simulink model "DWT_opt_fixed_point"  (R2022b)
settings: Solver=VariableStepAuto  StartTime=0.0  StopTime=st*279+st*length(signalx)  RelTol=1e-3
undefined symbols (not defined in the file): st, xc7z020clg484
libraries: hdlBasic x690, vmcUtilities x1
(part 3 of 3)

== system DWT_opt_fixed_point/axis_dwt/Syn_cell2/R_LO ==
  In1 : Inport
  AddSub{,1..6} (7 alike) : hdlBasic/AddSub  mode=Addition  use_carryin=off  use_carryout=off  en=off  latency=0  precision=User Defined  arith_type=Unsigned  n_bits=18  bin_pt=16  quantization=Truncate  overflow=Wrap  use_behavioral_HDL=off  hw_selection=Fabric  pipelined=off  XmcBlockStatus=1  maskContainerNames=tabcontainer1  block_type=addsub  block_config=sysgen:Addsub_config
  Constant : hdlBasic/Constant  const=0.23037781330885523  gui_display_data_type=Fixed-point  arith_type=Signed (2's comp)  n_bits=16  bin_pt=14  preci_type=Single  exp_width=8  frac_width=24  explicit_period=off  period=1  XmcBlockStatus=1  maskContainerNames=tabcontainer1  block_type=constant  block_config=sysgen:Constant_config
  Constant1 : hdlBasic/Constant  const=0.7148465705525415  gui_display_data_type=Fixed-point  arith_type=Signed (2's comp)  n_bits=16  bin_pt=14  preci_type=Single  exp_width=8  frac_width=24  explicit_period=off  period=1  XmcBlockStatus=1  maskContainerNames=tabcontainer1  block_type=constant  block_config=sysgen:Constant_config
  Constant2 : hdlBasic/Constant  const=0.6308807679295904  gui_display_data_type=Fixed-point  arith_type=Signed (2's comp)  n_bits=16  bin_pt=14  preci_type=Single  exp_width=8  frac_width=24  explicit_period=off  period=1  XmcBlockStatus=1  maskContainerNames=tabcontainer1  block_type=constant  block_config=sysgen:Constant_config
  Constant3 : hdlBasic/Constant  const=-0.02798376941698385  gui_display_data_type=Fixed-point  arith_type=Signed (2's comp)  n_bits=16  bin_pt=14  preci_type=Single  exp_width=8  frac_width=24  explicit_period=off  period=1  XmcBlockStatus=1  maskContainerNames=tabcontainer1  block_type=constant  block_config=sysgen:Constant_config
  Constant4 : hdlBasic/Constant  const=-0.18703481171888114  gui_display_data_type=Fixed-point  arith_type=Signed (2's comp)  n_bits=16  bin_pt=14  preci_type=Single  exp_width=8  frac_width=24  explicit_period=off  period=1  XmcBlockStatus=1  maskContainerNames=tabcontainer1  block_type=constant  block_config=sysgen:Constant_config
  Constant5 : hdlBasic/Constant  const=0.030841381835986965  gui_display_data_type=Fixed-point  arith_type=Signed (2's comp)  n_bits=16  bin_pt=14  preci_type=Single  exp_width=8  frac_width=24  explicit_period=off  period=1  XmcBlockStatus=1  maskContainerNames=tabcontainer1  block_type=constant  block_config=sysgen:Constant_config
  Constant6 : hdlBasic/Constant  const=0.032883011666982945  gui_display_data_type=Fixed-point  arith_type=Signed (2's comp)  n_bits=16  bin_pt=14  preci_type=Single  exp_width=8  frac_width=24  explicit_period=off  period=1  XmcBlockStatus=1  maskContainerNames=tabcontainer1  block_type=constant  block_config=sysgen:Constant_config
  Constant7 : hdlBasic/Constant  const=-0.010597401784997278  gui_display_data_type=Fixed-point  arith_type=Signed (2's comp)  n_bits=16  bin_pt=14  preci_type=Single  exp_width=8  frac_width=24  explicit_period=off  period=1  XmcBlockStatus=1  maskContainerNames=tabcontainer1  block_type=constant  block_config=sysgen:Constant_config
  Delay{,1..6} (7 alike) : hdlBasic/Delay  rst=off  en=off  latency=1  reg_retiming=off  XmcBlockStatus=1  maskContainerNames=group1  block_type=delay  block_config=sysgen:Delay_config
  Mult{,1..7} (8 alike) : hdlBasic/Mult  precision=User Defined  arith_type="Signed  (2's comp)"  n_bits=18  bin_pt=16  quantization=Truncate  overflow=Wrap  en=off  latency=0  use_behavioral_HDL=off  opt=Speed  use_embedded=on  optimum_pipeline=off  pipeline=on  use_rpm=on  placement_style=Triangular  XmcBlockStatus=1  maskContainerNames=group1  block_type=mult  block_config=sysgen:Mult_config  block_width=598  block_height=876
  Out1 : Outport
  wires:
  Delay3/1 -> Mult4/2, Delay4/1
  Mult2/1 -> AddSub1/1
  In1/1 -> Mult/2, Delay/1
  Constant6/1 -> Mult6/1
  Delay5/1 -> Mult6/2, Delay6/1
  Constant7/1 -> Mult7/1
  Delay1/1 -> Mult2/2, Delay2/1
  Delay/1 -> Mult1/2, Delay1/1
  AddSub6/1 -> Out1/1
  Delay2/1 -> Mult3/2, Delay3/1
  AddSub3/1 -> AddSub4/2
  Delay6/1 -> Mult7/2
  Mult3/1 -> AddSub2/1
  Constant5/1 -> Mult5/1
  AddSub/1 -> AddSub1/2
  Delay4/1 -> Mult5/2, Delay5/1
  Constant2/1 -> Mult2/1
  Mult7/1 -> AddSub6/1
  Mult1/1 -> AddSub/1
  Mult6/1 -> AddSub5/1
  AddSub4/1 -> AddSub5/2
  Mult4/1 -> AddSub3/1
  AddSub2/1 -> AddSub3/2
  Constant3/1 -> Mult3/1
  Constant/1 -> Mult/1
  Mult5/1 -> AddSub4/1
  AddSub1/1 -> AddSub2/2
  Constant4/1 -> Mult4/1
  Mult/1 -> AddSub/2
  AddSub5/1 -> AddSub6/2
  Constant1/1 -> Mult1/1

== system DWT_opt_fixed_point/axis_dwt/Syn_cell3/R_HI ==
  In1 : Inport
  AddSub{,1..6} (7 alike) : hdlBasic/AddSub  mode=Addition  use_carryin=off  use_carryout=off  en=off  latency=0  precision=User Defined  arith_type=Unsigned  n_bits=18  bin_pt=16  quantization=Truncate  overflow=Wrap  use_behavioral_HDL=off  hw_selection=Fabric  pipelined=off  XmcBlockStatus=1  maskContainerNames=tabcontainer1  block_type=addsub  block_config=sysgen:Addsub_config
  Constant : hdlBasic/Constant  const=-0.010597401784997278  gui_display_data_type=Fixed-point  arith_type=Signed (2's comp)  n_bits=16  bin_pt=14  preci_type=Single  exp_width=8  frac_width=24  explicit_period=off  period=1  XmcBlockStatus=1  maskContainerNames=tabcontainer1  block_type=constant  block_config=sysgen:Constant_config
  Constant1 : hdlBasic/Constant  const=-0.032883011666982945  gui_display_data_type=Fixed-point  arith_type=Signed (2's comp)  n_bits=16  bin_pt=14  preci_type=Single  exp_width=8  frac_width=24  explicit_period=off  period=1  XmcBlockStatus=1  maskContainerNames=tabcontainer1  block_type=constant  block_config=sysgen:Constant_config
  Constant2 : hdlBasic/Constant  const=0.030841381835986965  gui_display_data_type=Fixed-point  arith_type=Signed (2's comp)  n_bits=16  bin_pt=14  preci_type=Single  exp_width=8  frac_width=24  explicit_period=off  period=1  XmcBlockStatus=1  maskContainerNames=tabcontainer1  block_type=constant  block_config=sysgen:Constant_config
  Constant3 : hdlBasic/Constant  const=0.18703481171888114  gui_display_data_type=Fixed-point  arith_type=Signed (2's comp)  n_bits=16  bin_pt=14  preci_type=Single  exp_width=8  frac_width=24  explicit_period=off  period=1  XmcBlockStatus=1  maskContainerNames=tabcontainer1  block_type=constant  block_config=sysgen:Constant_config
  Constant4 : hdlBasic/Constant  const=-0.02798376941698385  gui_display_data_type=Fixed-point  arith_type=Signed (2's comp)  n_bits=16  bin_pt=14  preci_type=Single  exp_width=8  frac_width=24  explicit_period=off  period=1  XmcBlockStatus=1  maskContainerNames=tabcontainer1  block_type=constant  block_config=sysgen:Constant_config
  Constant5 : hdlBasic/Constant  const=-0.6308807679295904  gui_display_data_type=Fixed-point  arith_type=Signed (2's comp)  n_bits=16  bin_pt=14  preci_type=Single  exp_width=8  frac_width=24  explicit_period=off  period=1  XmcBlockStatus=1  maskContainerNames=tabcontainer1  block_type=constant  block_config=sysgen:Constant_config
  Constant6 : hdlBasic/Constant  const=0.7148465705525415  gui_display_data_type=Fixed-point  arith_type=Signed (2's comp)  n_bits=16  bin_pt=14  preci_type=Single  exp_width=8  frac_width=24  explicit_period=off  period=1  XmcBlockStatus=1  maskContainerNames=tabcontainer1  block_type=constant  block_config=sysgen:Constant_config
  Constant7 : hdlBasic/Constant  const=-0.23037781330885523  gui_display_data_type=Fixed-point  arith_type=Signed (2's comp)  n_bits=16  bin_pt=14  preci_type=Single  exp_width=8  frac_width=24  explicit_period=off  period=1  XmcBlockStatus=1  maskContainerNames=tabcontainer1  block_type=constant  block_config=sysgen:Constant_config
  Delay{,1..6} (7 alike) : hdlBasic/Delay  rst=off  en=off  latency=1  reg_retiming=off  XmcBlockStatus=1  maskContainerNames=group1  block_type=delay  block_config=sysgen:Delay_config
  Mult{,1..7} (8 alike) : hdlBasic/Mult  precision=User Defined  arith_type="Signed  (2's comp)"  n_bits=18  bin_pt=16  quantization=Truncate  overflow=Wrap  en=off  latency=0  use_behavioral_HDL=off  opt=Speed  use_embedded=on  optimum_pipeline=off  pipeline=on  use_rpm=on  placement_style=Triangular  XmcBlockStatus=1  maskContainerNames=group1  block_type=mult  block_config=sysgen:Mult_config  block_width=598  block_height=876
  Out1 : Outport
  wires:
  Delay3/1 -> Mult4/2, Delay4/1
  Mult2/1 -> AddSub1/1
  In1/1 -> Mult/2, Delay/1
  Constant6/1 -> Mult6/1
  Delay5/1 -> Mult6/2, Delay6/1
  Constant7/1 -> Mult7/1
  Delay1/1 -> Mult2/2, Delay2/1
  Delay/1 -> Mult1/2, Delay1/1
  AddSub6/1 -> Out1/1
  Delay2/1 -> Mult3/2, Delay3/1
  AddSub3/1 -> AddSub4/2
  Delay6/1 -> Mult7/2
  Mult3/1 -> AddSub2/1
  Constant5/1 -> Mult5/1
  AddSub/1 -> AddSub1/2
  Delay4/1 -> Mult5/2, Delay5/1
  Constant2/1 -> Mult2/1
  Mult7/1 -> AddSub6/1
  Mult1/1 -> AddSub/1
  Mult6/1 -> AddSub5/1
  AddSub4/1 -> AddSub5/2
  Mult4/1 -> AddSub3/1
  AddSub2/1 -> AddSub3/2
  Constant3/1 -> Mult3/1
  Constant/1 -> Mult/1
  Mult5/1 -> AddSub4/1
  AddSub1/1 -> AddSub2/2
  Constant4/1 -> Mult4/1
  Mult/1 -> AddSub/2
  AddSub5/1 -> AddSub6/2
  Constant1/1 -> Mult1/1

== system DWT_opt_fixed_point/axis_dwt/Syn_cell3/R_LO ==
  In1 : Inport
  AddSub{,1..6} (7 alike) : hdlBasic/AddSub  mode=Addition  use_carryin=off  use_carryout=off  en=off  latency=0  precision=User Defined  arith_type=Unsigned  n_bits=18  bin_pt=16  quantization=Truncate  overflow=Wrap  use_behavioral_HDL=off  hw_selection=Fabric  pipelined=off  XmcBlockStatus=1  maskContainerNames=tabcontainer1  block_type=addsub  block_config=sysgen:Addsub_config
  Constant : hdlBasic/Constant  const=0.23037781330885523  gui_display_data_type=Fixed-point  arith_type=Signed (2's comp)  n_bits=16  bin_pt=14  preci_type=Single  exp_width=8  frac_width=24  explicit_period=off  period=1  XmcBlockStatus=1  maskContainerNames=tabcontainer1  block_type=constant  block_config=sysgen:Constant_config
  Constant1 : hdlBasic/Constant  const=0.7148465705525415  gui_display_data_type=Fixed-point  arith_type=Signed (2's comp)  n_bits=16  bin_pt=14  preci_type=Single  exp_width=8  frac_width=24  explicit_period=off  period=1  XmcBlockStatus=1  maskContainerNames=tabcontainer1  block_type=constant  block_config=sysgen:Constant_config
  Constant2 : hdlBasic/Constant  const=0.6308807679295904  gui_display_data_type=Fixed-point  arith_type=Signed (2's comp)  n_bits=16  bin_pt=14  preci_type=Single  exp_width=8  frac_width=24  explicit_period=off  period=1  XmcBlockStatus=1  maskContainerNames=tabcontainer1  block_type=constant  block_config=sysgen:Constant_config
  Constant3 : hdlBasic/Constant  const=-0.02798376941698385  gui_display_data_type=Fixed-point  arith_type=Signed (2's comp)  n_bits=16  bin_pt=14  preci_type=Single  exp_width=8  frac_width=24  explicit_period=off  period=1  XmcBlockStatus=1  maskContainerNames=tabcontainer1  block_type=constant  block_config=sysgen:Constant_config
  Constant4 : hdlBasic/Constant  const=-0.18703481171888114  gui_display_data_type=Fixed-point  arith_type=Signed (2's comp)  n_bits=16  bin_pt=14  preci_type=Single  exp_width=8  frac_width=24  explicit_period=off  period=1  XmcBlockStatus=1  maskContainerNames=tabcontainer1  block_type=constant  block_config=sysgen:Constant_config
  Constant5 : hdlBasic/Constant  const=0.030841381835986965  gui_display_data_type=Fixed-point  arith_type=Signed (2's comp)  n_bits=16  bin_pt=14  preci_type=Single  exp_width=8  frac_width=24  explicit_period=off  period=1  XmcBlockStatus=1  maskContainerNames=tabcontainer1  block_type=constant  block_config=sysgen:Constant_config
  Constant6 : hdlBasic/Constant  const=0.032883011666982945  gui_display_data_type=Fixed-point  arith_type=Signed (2's comp)  n_bits=16  bin_pt=14  preci_type=Single  exp_width=8  frac_width=24  explicit_period=off  period=1  XmcBlockStatus=1  maskContainerNames=tabcontainer1  block_type=constant  block_config=sysgen:Constant_config
  Constant7 : hdlBasic/Constant  const=-0.010597401784997278  gui_display_data_type=Fixed-point  arith_type=Signed (2's comp)  n_bits=16  bin_pt=14  preci_type=Single  exp_width=8  frac_width=24  explicit_period=off  period=1  XmcBlockStatus=1  maskContainerNames=tabcontainer1  block_type=constant  block_config=sysgen:Constant_config
  Delay{,1..6} (7 alike) : hdlBasic/Delay  rst=off  en=off  latency=1  reg_retiming=off  XmcBlockStatus=1  maskContainerNames=group1  block_type=delay  block_config=sysgen:Delay_config
  Mult{,1..7} (8 alike) : hdlBasic/Mult  precision=User Defined  arith_type="Signed  (2's comp)"  n_bits=18  bin_pt=16  quantization=Truncate  overflow=Wrap  en=off  latency=0  use_behavioral_HDL=off  opt=Speed  use_embedded=on  optimum_pipeline=off  pipeline=on  use_rpm=on  placement_style=Triangular  XmcBlockStatus=1  maskContainerNames=group1  block_type=mult  block_config=sysgen:Mult_config  block_width=598  block_height=876
  Out1 : Outport
  wires:
  Delay3/1 -> Mult4/2, Delay4/1
  Mult2/1 -> AddSub1/1
  In1/1 -> Mult/2, Delay/1
  Constant6/1 -> Mult6/1
  Delay5/1 -> Mult6/2, Delay6/1
  Constant7/1 -> Mult7/1
  Delay1/1 -> Mult2/2, Delay2/1
  Delay/1 -> Mult1/2, Delay1/1
  AddSub6/1 -> Out1/1
  Delay2/1 -> Mult3/2, Delay3/1
  AddSub3/1 -> AddSub4/2
  Delay6/1 -> Mult7/2
  Mult3/1 -> AddSub2/1
  Constant5/1 -> Mult5/1
  AddSub/1 -> AddSub1/2
  Delay4/1 -> Mult5/2, Delay5/1
  Constant2/1 -> Mult2/1
  Mult7/1 -> AddSub6/1
  Mult1/1 -> AddSub/1
  Mult6/1 -> AddSub5/1
  AddSub4/1 -> AddSub5/2
  Mult4/1 -> AddSub3/1
  AddSub2/1 -> AddSub3/2
  Constant3/1 -> Mult3/1
  Constant/1 -> Mult/1
  Mult5/1 -> AddSub4/1
  AddSub1/1 -> AddSub2/2
  Constant4/1 -> Mult4/1
  Mult/1 -> AddSub/2
  AddSub5/1 -> AddSub6/2
  Constant1/1 -> Mult1/1

== system DWT_opt_fixed_point/axis_dwt/Syn_cell4/R_HI ==
  In1 : Inport
  AddSub{,1..6} (7 alike) : hdlBasic/AddSub  mode=Addition  use_carryin=off  use_carryout=off  en=off  latency=0  precision=User Defined  arith_type=Unsigned  n_bits=18  bin_pt=16  quantization=Truncate  overflow=Wrap  use_behavioral_HDL=off  hw_selection=Fabric  pipelined=off  XmcBlockStatus=1  maskContainerNames=tabcontainer1  block_type=addsub  block_config=sysgen:Addsub_config
  Constant : hdlBasic/Constant  const=-0.010597401784997278  gui_display_data_type=Fixed-point  arith_type=Signed (2's comp)  n_bits=16  bin_pt=14  preci_type=Single  exp_width=8  frac_width=24  explicit_period=off  period=1  XmcBlockStatus=1  maskContainerNames=tabcontainer1  block_type=constant  block_config=sysgen:Constant_config
  Constant1 : hdlBasic/Constant  const=-0.032883011666982945  gui_display_data_type=Fixed-point  arith_type=Signed (2's comp)  n_bits=16  bin_pt=14  preci_type=Single  exp_width=8  frac_width=24  explicit_period=off  period=1  XmcBlockStatus=1  maskContainerNames=tabcontainer1  block_type=constant  block_config=sysgen:Constant_config
  Constant2 : hdlBasic/Constant  const=0.030841381835986965  gui_display_data_type=Fixed-point  arith_type=Signed (2's comp)  n_bits=16  bin_pt=14  preci_type=Single  exp_width=8  frac_width=24  explicit_period=off  period=1  XmcBlockStatus=1  maskContainerNames=tabcontainer1  block_type=constant  block_config=sysgen:Constant_config
  Constant3 : hdlBasic/Constant  const=0.18703481171888114  gui_display_data_type=Fixed-point  arith_type=Signed (2's comp)  n_bits=16  bin_pt=14  preci_type=Single  exp_width=8  frac_width=24  explicit_period=off  period=1  XmcBlockStatus=1  maskContainerNames=tabcontainer1  block_type=constant  block_config=sysgen:Constant_config
  Constant4 : hdlBasic/Constant  const=-0.02798376941698385  gui_display_data_type=Fixed-point  arith_type=Signed (2's comp)  n_bits=16  bin_pt=14  preci_type=Single  exp_width=8  frac_width=24  explicit_period=off  period=1  XmcBlockStatus=1  maskContainerNames=tabcontainer1  block_type=constant  block_config=sysgen:Constant_config
  Constant5 : hdlBasic/Constant  const=-0.6308807679295904  gui_display_data_type=Fixed-point  arith_type=Signed (2's comp)  n_bits=16  bin_pt=14  preci_type=Single  exp_width=8  frac_width=24  explicit_period=off  period=1  XmcBlockStatus=1  maskContainerNames=tabcontainer1  block_type=constant  block_config=sysgen:Constant_config
  Constant6 : hdlBasic/Constant  const=0.7148465705525415  gui_display_data_type=Fixed-point  arith_type=Signed (2's comp)  n_bits=16  bin_pt=14  preci_type=Single  exp_width=8  frac_width=24  explicit_period=off  period=1  XmcBlockStatus=1  maskContainerNames=tabcontainer1  block_type=constant  block_config=sysgen:Constant_config
  Constant7 : hdlBasic/Constant  const=-0.23037781330885523  gui_display_data_type=Fixed-point  arith_type=Signed (2's comp)  n_bits=16  bin_pt=14  preci_type=Single  exp_width=8  frac_width=24  explicit_period=off  period=1  XmcBlockStatus=1  maskContainerNames=tabcontainer1  block_type=constant  block_config=sysgen:Constant_config
  Delay{,1..6} (7 alike) : hdlBasic/Delay  rst=off  en=off  latency=1  reg_retiming=off  XmcBlockStatus=1  maskContainerNames=group1  block_type=delay  block_config=sysgen:Delay_config
  Mult{,1..7} (8 alike) : hdlBasic/Mult  precision=User Defined  arith_type="Signed  (2's comp)"  n_bits=18  bin_pt=16  quantization=Truncate  overflow=Wrap  en=off  latency=0  use_behavioral_HDL=off  opt=Speed  use_embedded=on  optimum_pipeline=off  pipeline=on  use_rpm=on  placement_style=Triangular  XmcBlockStatus=1  maskContainerNames=group1  block_type=mult  block_config=sysgen:Mult_config  block_width=598  block_height=876
  Out1 : Outport
  wires:
  Delay3/1 -> Mult4/2, Delay4/1
  Mult2/1 -> AddSub1/1
  In1/1 -> Mult/2, Delay/1
  Constant6/1 -> Mult6/1
  Delay5/1 -> Mult6/2, Delay6/1
  Constant7/1 -> Mult7/1
  Delay1/1 -> Mult2/2, Delay2/1
  Delay/1 -> Mult1/2, Delay1/1
  AddSub6/1 -> Out1/1
  Delay2/1 -> Mult3/2, Delay3/1
  AddSub3/1 -> AddSub4/2
  Delay6/1 -> Mult7/2
  Mult3/1 -> AddSub2/1
  Constant5/1 -> Mult5/1
  AddSub/1 -> AddSub1/2
  Delay4/1 -> Mult5/2, Delay5/1
  Constant2/1 -> Mult2/1
  Mult7/1 -> AddSub6/1
  Mult1/1 -> AddSub/1
  Mult6/1 -> AddSub5/1
  AddSub4/1 -> AddSub5/2
  Mult4/1 -> AddSub3/1
  AddSub2/1 -> AddSub3/2
  Constant3/1 -> Mult3/1
  Constant/1 -> Mult/1
  Mult5/1 -> AddSub4/1
  AddSub1/1 -> AddSub2/2
  Constant4/1 -> Mult4/1
  Mult/1 -> AddSub/2
  AddSub5/1 -> AddSub6/2
  Constant1/1 -> Mult1/1

== system DWT_opt_fixed_point/axis_dwt/Syn_cell4/R_LO ==
  In1 : Inport
  AddSub{,1..6} (7 alike) : hdlBasic/AddSub  mode=Addition  use_carryin=off  use_carryout=off  en=off  latency=0  precision=User Defined  arith_type=Unsigned  n_bits=18  bin_pt=16  quantization=Truncate  overflow=Wrap  use_behavioral_HDL=off  hw_selection=Fabric  pipelined=off  XmcBlockStatus=1  maskContainerNames=tabcontainer1  block_type=addsub  block_config=sysgen:Addsub_config
  Constant : hdlBasic/Constant  const=0.23037781330885523  gui_display_data_type=Fixed-point  arith_type=Signed (2's comp)  n_bits=16  bin_pt=14  preci_type=Single  exp_width=8  frac_width=24  explicit_period=off  period=1  XmcBlockStatus=1  maskContainerNames=tabcontainer1  block_type=constant  block_config=sysgen:Constant_config
  Constant1 : hdlBasic/Constant  const=0.7148465705525415  gui_display_data_type=Fixed-point  arith_type=Signed (2's comp)  n_bits=16  bin_pt=14  preci_type=Single  exp_width=8  frac_width=24  explicit_period=off  period=1  XmcBlockStatus=1  maskContainerNames=tabcontainer1  block_type=constant  block_config=sysgen:Constant_config
  Constant2 : hdlBasic/Constant  const=0.6308807679295904  gui_display_data_type=Fixed-point  arith_type=Signed (2's comp)  n_bits=16  bin_pt=14  preci_type=Single  exp_width=8  frac_width=24  explicit_period=off  period=1  XmcBlockStatus=1  maskContainerNames=tabcontainer1  block_type=constant  block_config=sysgen:Constant_config
  Constant3 : hdlBasic/Constant  const=-0.02798376941698385  gui_display_data_type=Fixed-point  arith_type=Signed (2's comp)  n_bits=16  bin_pt=14  preci_type=Single  exp_width=8  frac_width=24  explicit_period=off  period=1  XmcBlockStatus=1  maskContainerNames=tabcontainer1  block_type=constant  block_config=sysgen:Constant_config
  Constant4 : hdlBasic/Constant  const=-0.18703481171888114  gui_display_data_type=Fixed-point  arith_type=Signed (2's comp)  n_bits=16  bin_pt=14  preci_type=Single  exp_width=8  frac_width=24  explicit_period=off  period=1  XmcBlockStatus=1  maskContainerNames=tabcontainer1  block_type=constant  block_config=sysgen:Constant_config
  Constant5 : hdlBasic/Constant  const=0.030841381835986965  gui_display_data_type=Fixed-point  arith_type=Signed (2's comp)  n_bits=16  bin_pt=14  preci_type=Single  exp_width=8  frac_width=24  explicit_period=off  period=1  XmcBlockStatus=1  maskContainerNames=tabcontainer1  block_type=constant  block_config=sysgen:Constant_config
  Constant6 : hdlBasic/Constant  const=0.032883011666982945  gui_display_data_type=Fixed-point  arith_type=Signed (2's comp)  n_bits=16  bin_pt=14  preci_type=Single  exp_width=8  frac_width=24  explicit_period=off  period=1  XmcBlockStatus=1  maskContainerNames=tabcontainer1  block_type=constant  block_config=sysgen:Constant_config
  Constant7 : hdlBasic/Constant  const=-0.010597401784997278  gui_display_data_type=Fixed-point  arith_type=Signed (2's comp)  n_bits=16  bin_pt=14  preci_type=Single  exp_width=8  frac_width=24  explicit_period=off  period=1  XmcBlockStatus=1  maskContainerNames=tabcontainer1  block_type=constant  block_config=sysgen:Constant_config
  Delay{,1..6} (7 alike) : hdlBasic/Delay  rst=off  en=off  latency=1  reg_retiming=off  XmcBlockStatus=1  maskContainerNames=group1  block_type=delay  block_config=sysgen:Delay_config
  Mult{,1..7} (8 alike) : hdlBasic/Mult  precision=User Defined  arith_type="Signed  (2's comp)"  n_bits=18  bin_pt=16  quantization=Truncate  overflow=Wrap  en=off  latency=0  use_behavioral_HDL=off  opt=Speed  use_embedded=on  optimum_pipeline=off  pipeline=on  use_rpm=on  placement_style=Triangular  XmcBlockStatus=1  maskContainerNames=group1  block_type=mult  block_config=sysgen:Mult_config  block_width=598  block_height=876
  Out1 : Outport
  wires:
  Delay3/1 -> Mult4/2, Delay4/1
  Mult2/1 -> AddSub1/1
  In1/1 -> Mult/2, Delay/1
  Constant6/1 -> Mult6/1
  Delay5/1 -> Mult6/2, Delay6/1
  Constant7/1 -> Mult7/1
  Delay1/1 -> Mult2/2, Delay2/1
  Delay/1 -> Mult1/2, Delay1/1
  AddSub6/1 -> Out1/1
  Delay2/1 -> Mult3/2, Delay3/1
  AddSub3/1 -> AddSub4/2
  Delay6/1 -> Mult7/2
  Mult3/1 -> AddSub2/1
  Constant5/1 -> Mult5/1
  AddSub/1 -> AddSub1/2
  Delay4/1 -> Mult5/2, Delay5/1
  Constant2/1 -> Mult2/1
  Mult7/1 -> AddSub6/1
  Mult1/1 -> AddSub/1
  Mult6/1 -> AddSub5/1
  AddSub4/1 -> AddSub5/2
  Mult4/1 -> AddSub3/1
  AddSub2/1 -> AddSub3/2
  Constant3/1 -> Mult3/1
  Constant/1 -> Mult/1
  Mult5/1 -> AddSub4/1
  AddSub1/1 -> AddSub2/2
  Constant4/1 -> Mult4/1
  Mult/1 -> AddSub/2
  AddSub5/1 -> AddSub6/2
  Constant1/1 -> Mult1/1

== system DWT_opt_fixed_point/axis_dwt/Syn_cell5/R_HI ==
  In1 : Inport
  AddSub{,1..6} (7 alike) : hdlBasic/AddSub  mode=Addition  use_carryin=off  use_carryout=off  en=off  latency=0  precision=User Defined  arith_type=Unsigned  n_bits=18  bin_pt=16  quantization=Truncate  overflow=Wrap  use_behavioral_HDL=off  hw_selection=Fabric  pipelined=off  XmcBlockStatus=1  maskContainerNames=tabcontainer1  block_type=addsub  block_config=sysgen:Addsub_config
  Constant : hdlBasic/Constant  const=-0.010597401784997278  gui_display_data_type=Fixed-point  arith_type=Signed (2's comp)  n_bits=16  bin_pt=14  preci_type=Single  exp_width=8  frac_width=24  explicit_period=off  period=1  XmcBlockStatus=1  maskContainerNames=tabcontainer1  block_type=constant  block_config=sysgen:Constant_config
  Constant1 : hdlBasic/Constant  const=-0.032883011666982945  gui_display_data_type=Fixed-point  arith_type=Signed (2's comp)  n_bits=16  bin_pt=14  preci_type=Single  exp_width=8  frac_width=24  explicit_period=off  period=1  XmcBlockStatus=1  maskContainerNames=tabcontainer1  block_type=constant  block_config=sysgen:Constant_config
  Constant2 : hdlBasic/Constant  const=0.030841381835986965  gui_display_data_type=Fixed-point  arith_type=Signed (2's comp)  n_bits=16  bin_pt=14  preci_type=Single  exp_width=8  frac_width=24  explicit_period=off  period=1  XmcBlockStatus=1  maskContainerNames=tabcontainer1  block_type=constant  block_config=sysgen:Constant_config
  Constant3 : hdlBasic/Constant  const=0.18703481171888114  gui_display_data_type=Fixed-point  arith_type=Signed (2's comp)  n_bits=16  bin_pt=14  preci_type=Single  exp_width=8  frac_width=24  explicit_period=off  period=1  XmcBlockStatus=1  maskContainerNames=tabcontainer1  block_type=constant  block_config=sysgen:Constant_config
  Constant4 : hdlBasic/Constant  const=-0.02798376941698385  gui_display_data_type=Fixed-point  arith_type=Signed (2's comp)  n_bits=16  bin_pt=14  preci_type=Single  exp_width=8  frac_width=24  explicit_period=off  period=1  XmcBlockStatus=1  maskContainerNames=tabcontainer1  block_type=constant  block_config=sysgen:Constant_config
  Constant5 : hdlBasic/Constant  const=-0.6308807679295904  gui_display_data_type=Fixed-point  arith_type=Signed (2's comp)  n_bits=16  bin_pt=14  preci_type=Single  exp_width=8  frac_width=24  explicit_period=off  period=1  XmcBlockStatus=1  maskContainerNames=tabcontainer1  block_type=constant  block_config=sysgen:Constant_config
  Constant6 : hdlBasic/Constant  const=0.7148465705525415  gui_display_data_type=Fixed-point  arith_type=Signed (2's comp)  n_bits=16  bin_pt=14  preci_type=Single  exp_width=8  frac_width=24  explicit_period=off  period=1  XmcBlockStatus=1  maskContainerNames=tabcontainer1  block_type=constant  block_config=sysgen:Constant_config
  Constant7 : hdlBasic/Constant  const=-0.23037781330885523  gui_display_data_type=Fixed-point  arith_type=Signed (2's comp)  n_bits=16  bin_pt=14  preci_type=Single  exp_width=8  frac_width=24  explicit_period=off  period=1  XmcBlockStatus=1  maskContainerNames=tabcontainer1  block_type=constant  block_config=sysgen:Constant_config
  Delay{,1..6} (7 alike) : hdlBasic/Delay  rst=off  en=off  latency=1  reg_retiming=off  XmcBlockStatus=1  maskContainerNames=group1  block_type=delay  block_config=sysgen:Delay_config
  Mult{,1..7} (8 alike) : hdlBasic/Mult  precision=User Defined  arith_type="Signed  (2's comp)"  n_bits=18  bin_pt=16  quantization=Truncate  overflow=Wrap  en=off  latency=0  use_behavioral_HDL=off  opt=Speed  use_embedded=on  optimum_pipeline=off  pipeline=on  use_rpm=on  placement_style=Triangular  XmcBlockStatus=1  maskContainerNames=group1  block_type=mult  block_config=sysgen:Mult_config  block_width=598  block_height=876
  Out1 : Outport
  wires:
  Delay3/1 -> Mult4/2, Delay4/1
  Mult2/1 -> AddSub1/1
  In1/1 -> Mult/2, Delay/1
  Constant6/1 -> Mult6/1
  Delay5/1 -> Mult6/2, Delay6/1
  Constant7/1 -> Mult7/1
  Delay1/1 -> Mult2/2, Delay2/1
  Delay/1 -> Mult1/2, Delay1/1
  AddSub6/1 -> Out1/1
  Delay2/1 -> Mult3/2, Delay3/1
  AddSub3/1 -> AddSub4/2
  Delay6/1 -> Mult7/2
  Mult3/1 -> AddSub2/1
  Constant5/1 -> Mult5/1
  AddSub/1 -> AddSub1/2
  Delay4/1 -> Mult5/2, Delay5/1
  Constant2/1 -> Mult2/1
  Mult7/1 -> AddSub6/1
  Mult1/1 -> AddSub/1
  Mult6/1 -> AddSub5/1
  AddSub4/1 -> AddSub5/2
  Mult4/1 -> AddSub3/1
  AddSub2/1 -> AddSub3/2
  Constant3/1 -> Mult3/1
  Constant/1 -> Mult/1
  Mult5/1 -> AddSub4/1
  AddSub1/1 -> AddSub2/2
  Constant4/1 -> Mult4/1
  Mult/1 -> AddSub/2
  AddSub5/1 -> AddSub6/2
  Constant1/1 -> Mult1/1

== system DWT_opt_fixed_point/axis_dwt/Syn_cell5/R_LO ==
  In1 : Inport
  AddSub{,1..6} (7 alike) : hdlBasic/AddSub  mode=Addition  use_carryin=off  use_carryout=off  en=off  latency=0  precision=User Defined  arith_type=Unsigned  n_bits=18  bin_pt=16  quantization=Truncate  overflow=Wrap  use_behavioral_HDL=off  hw_selection=Fabric  pipelined=off  XmcBlockStatus=1  maskContainerNames=tabcontainer1  block_type=addsub  block_config=sysgen:Addsub_config
  Constant : hdlBasic/Constant  const=0.23037781330885523  gui_display_data_type=Fixed-point  arith_type=Signed (2's comp)  n_bits=16  bin_pt=14  preci_type=Single  exp_width=8  frac_width=24  explicit_period=off  period=1  XmcBlockStatus=1  maskContainerNames=tabcontainer1  block_type=constant  block_config=sysgen:Constant_config
  Constant1 : hdlBasic/Constant  const=0.7148465705525415  gui_display_data_type=Fixed-point  arith_type=Signed (2's comp)  n_bits=16  bin_pt=14  preci_type=Single  exp_width=8  frac_width=24  explicit_period=off  period=1  XmcBlockStatus=1  maskContainerNames=tabcontainer1  block_type=constant  block_config=sysgen:Constant_config
  Constant2 : hdlBasic/Constant  const=0.6308807679295904  gui_display_data_type=Fixed-point  arith_type=Signed (2's comp)  n_bits=16  bin_pt=14  preci_type=Single  exp_width=8  frac_width=24  explicit_period=off  period=1  XmcBlockStatus=1  maskContainerNames=tabcontainer1  block_type=constant  block_config=sysgen:Constant_config
  Constant3 : hdlBasic/Constant  const=-0.02798376941698385  gui_display_data_type=Fixed-point  arith_type=Signed (2's comp)  n_bits=16  bin_pt=14  preci_type=Single  exp_width=8  frac_width=24  explicit_period=off  period=1  XmcBlockStatus=1  maskContainerNames=tabcontainer1  block_type=constant  block_config=sysgen:Constant_config
  Constant4 : hdlBasic/Constant  const=-0.18703481171888114  gui_display_data_type=Fixed-point  arith_type=Signed (2's comp)  n_bits=16  bin_pt=14  preci_type=Single  exp_width=8  frac_width=24  explicit_period=off  period=1  XmcBlockStatus=1  maskContainerNames=tabcontainer1  block_type=constant  block_config=sysgen:Constant_config
  Constant5 : hdlBasic/Constant  const=0.030841381835986965  gui_display_data_type=Fixed-point  arith_type=Signed (2's comp)  n_bits=16  bin_pt=14  preci_type=Single  exp_width=8  frac_width=24  explicit_period=off  period=1  XmcBlockStatus=1  maskContainerNames=tabcontainer1  block_type=constant  block_config=sysgen:Constant_config
  Constant6 : hdlBasic/Constant  const=0.032883011666982945  gui_display_data_type=Fixed-point  arith_type=Signed (2's comp)  n_bits=16  bin_pt=14  preci_type=Single  exp_width=8  frac_width=24  explicit_period=off  period=1  XmcBlockStatus=1  maskContainerNames=tabcontainer1  block_type=constant  block_config=sysgen:Constant_config
  Constant7 : hdlBasic/Constant  const=-0.010597401784997278  gui_display_data_type=Fixed-point  arith_type=Signed (2's comp)  n_bits=16  bin_pt=14  preci_type=Single  exp_width=8  frac_width=24  explicit_period=off  period=1  XmcBlockStatus=1  maskContainerNames=tabcontainer1  block_type=constant  block_config=sysgen:Constant_config
  Delay{,1..6} (7 alike) : hdlBasic/Delay  rst=off  en=off  latency=1  reg_retiming=off  XmcBlockStatus=1  maskContainerNames=group1  block_type=delay  block_config=sysgen:Delay_config
  Mult{,1..7} (8 alike) : hdlBasic/Mult  precision=User Defined  arith_type="Signed  (2's comp)"  n_bits=18  bin_pt=16  quantization=Truncate  overflow=Wrap  en=off  latency=0  use_behavioral_HDL=off  opt=Speed  use_embedded=on  optimum_pipeline=off  pipeline=on  use_rpm=on  placement_style=Triangular  XmcBlockStatus=1  maskContainerNames=group1  block_type=mult  block_config=sysgen:Mult_config  block_width=598  block_height=876
  Out1 : Outport
  wires:
  Delay3/1 -> Mult4/2, Delay4/1
  Mult2/1 -> AddSub1/1
  In1/1 -> Mult/2, Delay/1
  Constant6/1 -> Mult6/1
  Delay5/1 -> Mult6/2, Delay6/1
  Constant7/1 -> Mult7/1
  Delay1/1 -> Mult2/2, Delay2/1
  Delay/1 -> Mult1/2, Delay1/1
  AddSub6/1 -> Out1/1
  Delay2/1 -> Mult3/2, Delay3/1
  AddSub3/1 -> AddSub4/2
  Delay6/1 -> Mult7/2
  Mult3/1 -> AddSub2/1
  Constant5/1 -> Mult5/1
  AddSub/1 -> AddSub1/2
  Delay4/1 -> Mult5/2, Delay5/1
  Constant2/1 -> Mult2/1
  Mult7/1 -> AddSub6/1
  Mult1/1 -> AddSub/1
  Mult6/1 -> AddSub5/1
  AddSub4/1 -> AddSub5/2
  Mult4/1 -> AddSub3/1
  AddSub2/1 -> AddSub3/2
  Constant3/1 -> Mult3/1
  Constant/1 -> Mult/1
  Mult5/1 -> AddSub4/1
  AddSub1/1 -> AddSub2/2
  Constant4/1 -> Mult4/1
  Mult/1 -> AddSub/2
  AddSub5/1 -> AddSub6/2
  Constant1/1 -> Mult1/1
